simulink model "Swarm_Robot_Final"  (R2020b)
settings: Solver=FixedStepAuto  StartTime=0.0  StopTime=inf  FixedStep=sampleTime  RelTol=1e-3
PreLoadFcn:
  | % Simulation parameters
  | load exampleMap
  | sampleTime = 0.05;
  | 
  | % Robot parameters
  | wheelRadius = 0.025;
  | robotRadius = 0.35;
  | 
  | % Lidar parameters
  | sensorOffset = [0,0];
  | scanAngles = linspace(-pi/2,pi/2,9)';
  | maxRange = 5;
libraries: mobileRoboticsLib x10
settings Model: EnablePacing=on  Creator=scastro  LastModifiedBy=Ashish Sharma
settings DataIOCC: ReturnWorkspaceOutputs=off
settings DebuggingCC: PregeneratedLibrarySubsystemCodeDiagnostic=none  ArithmeticOperatorsInVariantConditions=warning
settings SFSimCC: SimUseLocalCustomCode=off  CustomCodeUndefinedFunction=UseInterfaceOnly
settings RTWCC: RTWUseLocalCustomCode=off

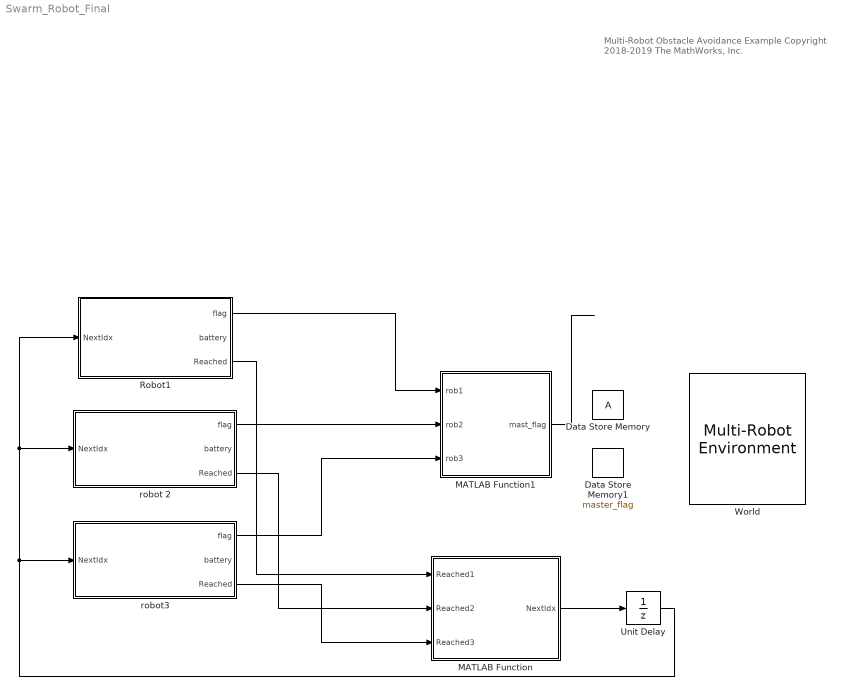
== system Swarm_Robot_Final ==
  note: Multi-Robot Obstacle
      | Avoidance Example
      |
      | Copyright 2018-2019 The MathWorks, Inc.
  Data Store Memory : DataStoreMemory  ReadBeforeWriteMsg=warning  WriteAfterWriteMsg=warning  WriteAfterReadMsg=warning  InitialValue=[1000 1000 1000]  ShowAdditionalParam=off  OutDataTypeStr=double
  Data Store Memory1 : DataStoreMemory  DataStoreName=master_flag  ReadBeforeWriteMsg=warning  WriteAfterWriteMsg=warning  WriteAfterReadMsg=warning  ShowAdditionalParam=off  OutDataTypeStr=double
  MATLAB Function : MATLAB Function  TreatAsAtomicUnit=on
  MATLAB Function1 : MATLAB Function  TreatAsAtomicUnit=on
  "Robot1 " : Subsystem
  Unit Delay : UnitDelay  SampleTime=-1  HasFrameUpgradeWarning=on
  World : mobileRoboticsLib/Environments/Multi-Robot Environment  numRobots=3  showWaypoints=off  showObjects=off  objectColors=[1 0 0;0 1 0;0 0 1]  objectMarkers='s'  showRobotIds=on  plotSensorLines=on
      settings: SourceProductName=Mobile Robotics Simulation Toolbox
  robot 2 : Subsystem
  robot3 : Subsystem
  wires:
  "Robot1 "/1(flag) -> MATLAB Function1/1(rob1)
  robot 2/1(flag) -> MATLAB Function1/2(rob2)
  robot3/1(flag) -> MATLAB Function1/3(rob3)
  "Robot1 "/3(Reached) -> MATLAB Function/1(Reached1)
  MATLAB Function/1(NextIdx) -> Unit Delay/1
  Unit Delay/1 -> "Robot1 "/1(NextIdx), robot 2/1(NextIdx), robot3/1(NextIdx)
  robot 2/3(Reached) -> MATLAB Function/2(Reached2)
  robot3/3(Reached) -> MATLAB Function/3(Reached3)
  MATLAB Function1/1(mast_flag) -> ?

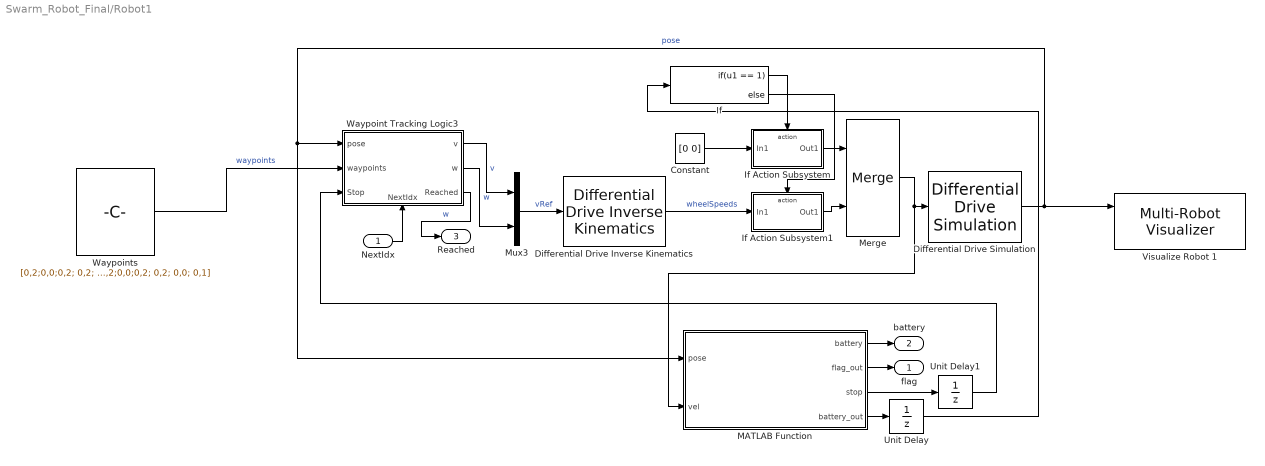
== system Swarm_Robot_Final/Robot1  ==
  NextIdx : Inport
  Constant : Constant  Value=[0 0]
  Differential Drive Inverse Kinematics : mobileRoboticsLib/Kinematic Models/Differential Drive/Differential Drive Inverse Kinematics  wheelRadius=R  wheelBase=L
      settings: SourceProductName=Mobile Robotics Simulation Toolbox
  Differential Drive Simulation : mobileRoboticsLib/Kinematic Models/Differential Drive/Differential Drive Simulation  wheelRadius=R  wheelBase=L  initX=0  initY=2  initAngle=0  Ts=sampleTime
      settings: SourceProductName=Mobile Robotics Simulation Toolbox
  If : If  IfExpression=u1 == 1
  If Action Subsystem : Subsystem  TreatAsAtomicUnit=on
  If Action Subsystem1 : Subsystem  TreatAsAtomicUnit=on
  MATLAB Function : MATLAB Function  TreatAsAtomicUnit=on
  Merge : Merge
  Mux3 : Mux  Inputs=2
  Unit Delay : UnitDelay  SampleTime=-1  HasFrameUpgradeWarning=on
  Unit Delay1 : UnitDelay  SampleTime=-1  HasFrameUpgradeWarning=on
  Visualize Robot 1 : mobileRoboticsLib/Environments/Multi-Robot Visualizer  idx=1  radius=robotRadius  robotColor=[0 0 1]  showTraj=off  hasLidar=on  sensorOffset=sensorOffset  scanAngles=scanAngles  maxNumScans=0  hasObjDetector=off  objDetectorOffset=[0,0]  objDetectorAngle=0  objDetectorFOV=pi/2  objDetectorMaxRange=5  hasRobotDetector=off  robotDetectorOffset=[0,0]  robotDetectorAngle=0  robotDetectorFOV=pi/3  robotDetectorMaxRange=5  robotDetectorNumDetections=0
      settings: SourceProductName=Mobile Robotics Simulation Toolbox
  Waypoint Tracking Logic3 : Stateflow chart  TreatAsAtomicUnit=on
      settings: PortSchema="{\"entries\":[{\"content\":{\"sides\":[{\"content\":{\"connectorIds\":[\"In1\",\"In2\",\"In3\"]},\"type\":\"ConnectorPlacement.EquallySpacedRectSide\",\"uuid\":\"0f37e2f5-7e3e-44b4-b5ad-f9c608efa7e9\"},{\"content\":{\"connectorIds\":[\"Out1\",\"Out2\",\"Out3\"],\"side\":\"RIGHT\"},\"type\":\"ConnectorPlacement.EquallySpacedRectSide\",\"uuid\":\"845bf79f-ea31-423e-b1b0-9ff668e9d8f6\"},{\"content\":{\"connectorIds\":[],\"side\":\"TOP\"},\"type\":\"ConnectorPlacement.EquallySpacedRectSide\",\"uuid\":\"8bec6743-f757-46fc-95b1-a88bb4057338\"},{\"content\":{\"connectorIds\":[\"In4\"],\"side\":\"BOTTOM\"},\"type\":\"ConnectorPlacement.EquallySpacedRectSide\",\"uuid\":\"241e6e67-ff0c-43d0-b4d4-f7a4fa1e9b40\"},{\"content\":{\"connectorIds\":[],\"side\":\"HIDDEN\"},\"type\":\"ConnectorPlacement.EquallySpacedRectSide\",\"uuid\":\"709a4cd5-ab66-4303-a1be-0f54eaafc229\"}]},\"type\":\"ConnectorPlacement.EquallySpacedConnector\",\"uuid\":\"0437a356-16a4-4e9a-ad43-fdf8419276a1\"}],\"packageUris\":[\"http://schema.mathworks.com/mf0/Connector/R2020b\"],\"version\":\"1.0\"}"
  Waypoints : Constant  Value=[0,2;0,0;0,2; 0,2; 0,0; 0,1;0,2;0,0;0,2; 0,2; 0,0; 0,1;0,2;0,0;0,2; 0,2; 0,0; 0,1]
  flag : Outport
  battery : Outport  Port=2
  Reached : Outport  Port=3
  wires:
  Waypoints/1 -> Waypoint Tracking Logic3/2(waypoints)  "waypoints"
  MATLAB Function/1(battery) -> battery/1
  Differential Drive Simulation/1 -> Visualize Robot 1/1, MATLAB Function/1(pose), Waypoint Tracking Logic3/1(pose)  "pose"
  Merge/1 -> MATLAB Function/2(vel), Differential Drive Simulation/1
  Mux3/1 -> Differential Drive Inverse Kinematics/1  "vRef"
  MATLAB Function/2(flag_out) -> flag/1
  If/1 -> If Action Subsystem/Action
  If/2 -> If Action Subsystem1/Action
  Constant/1 -> If Action Subsystem/1(In1)
  If Action Subsystem1/1(Out1) -> Merge/2
  If Action Subsystem/1(Out1) -> Merge/1
  Waypoint Tracking Logic3/1(v) -> Mux3/1  "v"
  Differential Drive Inverse Kinematics/1 -> If Action Subsystem1/1(In1)  "wheelSpeeds"
  Waypoint Tracking Logic3/2(w) -> Mux3/2  "w"
  NextIdx/1 -> Waypoint Tracking Logic3/4(NextIdx)
  Waypoint Tracking Logic3/3(Reached) -> Reached/1  "w"
  MATLAB Function/4(battery_out) -> Unit Delay/1
  Unit Delay/1 -> If/1
  MATLAB Function/3(stop) -> Unit Delay1/1
  Unit Delay1/1 -> Waypoint Tracking Logic3/3(Stop)

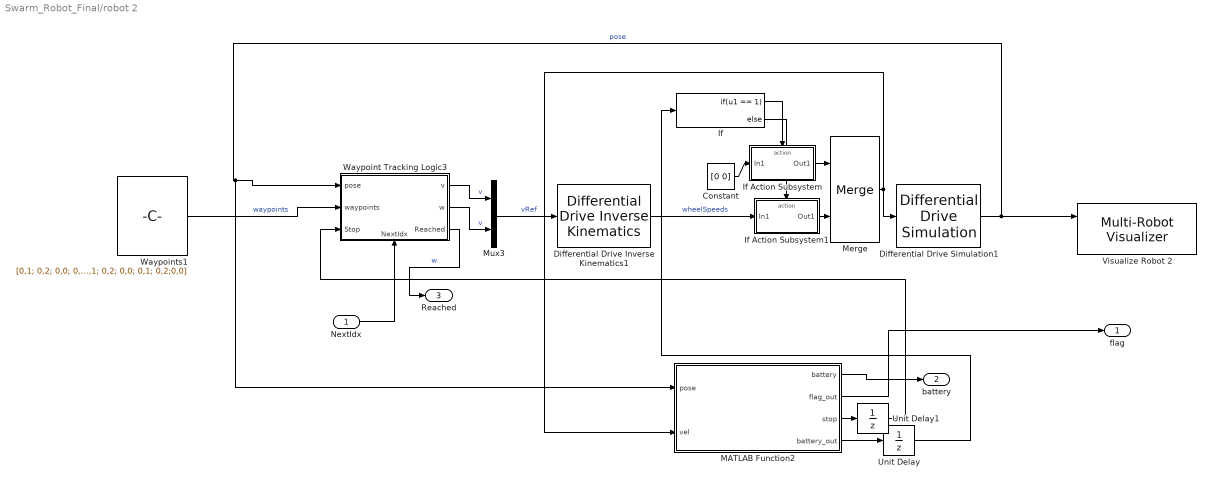
== system Swarm_Robot_Final/robot 2 ==
  NextIdx : Inport
  Constant : Constant  Value=[0 0]
  Differential Drive Inverse Kinematics1 : mobileRoboticsLib/Kinematic Models/Differential Drive/Differential Drive Inverse Kinematics  wheelRadius=R  wheelBase=L
      settings: SourceProductName=Mobile Robotics Simulation Toolbox
  Differential Drive Simulation1 : mobileRoboticsLib/Kinematic Models/Differential Drive/Differential Drive Simulation  wheelRadius=R  wheelBase=L  initX=0  initY=1  initAngle=0  Ts=sampleTime
      settings: SourceProductName=Mobile Robotics Simulation Toolbox
  If : If  IfExpression=u1 == 1
  If Action Subsystem : Subsystem  TreatAsAtomicUnit=on
  If Action Subsystem1 : Subsystem  TreatAsAtomicUnit=on
  MATLAB Function2 : MATLAB Function  TreatAsAtomicUnit=on
  Merge : Merge
  Mux3 : Mux  Inputs=2
  Unit Delay : UnitDelay  SampleTime=-1  HasFrameUpgradeWarning=on
  Unit Delay1 : UnitDelay  SampleTime=-1  HasFrameUpgradeWarning=on
  Visualize Robot 2 : mobileRoboticsLib/Environments/Multi-Robot Visualizer  idx=2  radius=robotRadius  robotColor=[0 0 1]  showTraj=off  hasLidar=on  sensorOffset=sensorOffset  scanAngles=scanAngles  maxNumScans=0  hasObjDetector=off  objDetectorOffset=[0 0]  objDetectorAngle=0  objDetectorFOV=pi/2  objDetectorMaxRange=5  hasRobotDetector=off  robotDetectorOffset=[0,0]  robotDetectorAngle=0  robotDetectorFOV=pi/3  robotDetectorMaxRange=5  robotDetectorNumDetections=0
      settings: SourceProductName=Mobile Robotics Simulation Toolbox
  Waypoint Tracking Logic3 : Stateflow chart  TreatAsAtomicUnit=on
      settings: PortSchema="{\"entries\":[{\"content\":{\"sides\":[{\"content\":{\"connectorIds\":[\"In1\",\"In2\",\"In3\"]},\"type\":\"ConnectorPlacement.EquallySpacedRectSide\",\"uuid\":\"0f37e2f5-7e3e-44b4-b5ad-f9c608efa7e9\"},{\"content\":{\"connectorIds\":[\"Out1\",\"Out2\",\"Out3\"],\"side\":\"RIGHT\"},\"type\":\"ConnectorPlacement.EquallySpacedRectSide\",\"uuid\":\"845bf79f-ea31-423e-b1b0-9ff668e9d8f6\"},{\"content\":{\"connectorIds\":[],\"side\":\"TOP\"},\"type\":\"ConnectorPlacement.EquallySpacedRectSide\",\"uuid\":\"8bec6743-f757-46fc-95b1-a88bb4057338\"},{\"content\":{\"connectorIds\":[\"In4\"],\"side\":\"BOTTOM\"},\"type\":\"ConnectorPlacement.EquallySpacedRectSide\",\"uuid\":\"241e6e67-ff0c-43d0-b4d4-f7a4fa1e9b40\"},{\"content\":{\"connectorIds\":[],\"side\":\"HIDDEN\"},\"type\":\"ConnectorPlacement.EquallySpacedRectSide\",\"uuid\":\"709a4cd5-ab66-4303-a1be-0f54eaafc229\"}]},\"type\":\"ConnectorPlacement.EquallySpacedConnector\",\"uuid\":\"0437a356-16a4-4e9a-ad43-fdf8419276a1\"}],\"packageUris\":[\"http://schema.mathworks.com/mf0/Connector/R2020b\"],\"version\":\"1.0\"}"
  Waypoints1 : Constant  Value=[0,1; 0,2; 0,0; 0,1; 0,2;0,0;0,1; 0,2; 0,0; 0,1; 0,2;0,0;0,1; 0,2; 0,0; 0,1; 0,2;0,0]
  flag : Outport
  battery : Outport  Port=2
  Reached : Outport  Port=3
  wires:
  MATLAB Function2/2(flag_out) -> flag/1
  Differential Drive Inverse Kinematics1/1 -> If Action Subsystem1/1(In1)  "wheelSpeeds"
  Mux3/1 -> Differential Drive Inverse Kinematics1/1  "vRef"
  Waypoints1/1 -> Waypoint Tracking Logic3/2(waypoints)  "waypoints"
  Differential Drive Simulation1/1 -> MATLAB Function2/1(pose), Waypoint Tracking Logic3/1(pose), Visualize Robot 2/1  "pose"
  MATLAB Function2/1(battery) -> battery/1
  If Action Subsystem1/1(Out1) -> Merge/2
  If/2 -> If Action Subsystem1/Action
  Constant/1 -> If Action Subsystem/1(In1)
  If/1 -> If Action Subsystem/Action
  If Action Subsystem/1(Out1) -> Merge/1
  Merge/1 -> Differential Drive Simulation1/1, MATLAB Function2/2(vel)
  NextIdx/1 -> Waypoint Tracking Logic3/4(NextIdx)
  Waypoint Tracking Logic3/1(v) -> Mux3/1  "v"
  Waypoint Tracking Logic3/2(w) -> Mux3/2  "v"
  Waypoint Tracking Logic3/3(Reached) -> Reached/1  "w"
  MATLAB Function2/4(battery_out) -> Unit Delay/1
  Unit Delay/1 -> If/1
  MATLAB Function2/3(stop) -> Unit Delay1/1
  Unit Delay1/1 -> Waypoint Tracking Logic3/3(Stop)

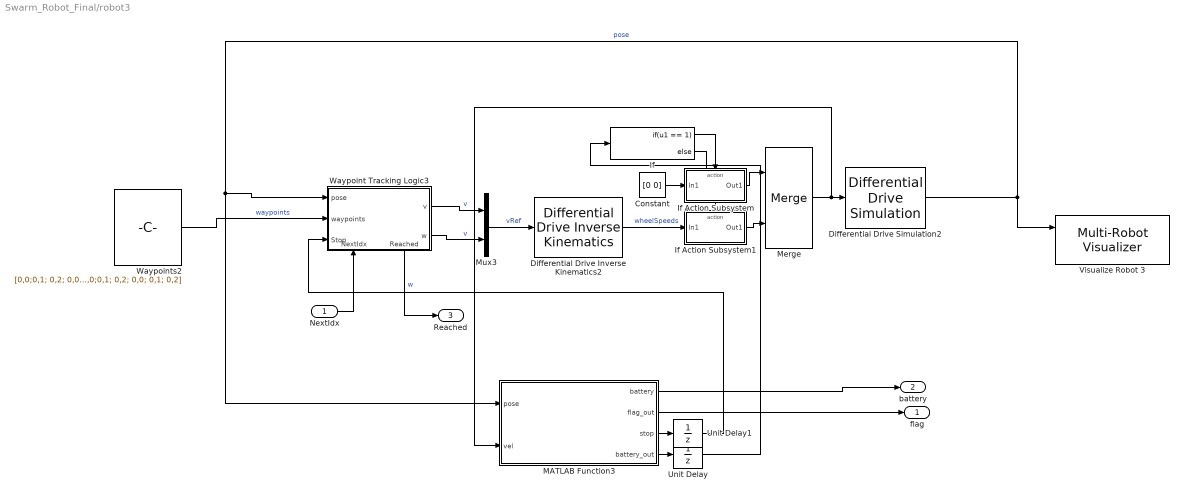
== system Swarm_Robot_Final/robot3 ==
  NextIdx : Inport
  Constant : Constant  Value=[0 0]
  Differential Drive Inverse Kinematics2 : mobileRoboticsLib/Kinematic Models/Differential Drive/Differential Drive Inverse Kinematics  wheelRadius=R  wheelBase=L
      settings: SourceProductName=Mobile Robotics Simulation Toolbox
  Differential Drive Simulation2 : mobileRoboticsLib/Kinematic Models/Differential Drive/Differential Drive Simulation  wheelRadius=R  wheelBase=L  initX=0  initY=0  initAngle=0  Ts=sampleTime
      settings: SourceProductName=Mobile Robotics Simulation Toolbox
  If : If  IfExpression=u1 == 1
  If Action Subsystem : Subsystem  TreatAsAtomicUnit=on
  If Action Subsystem1 : Subsystem  TreatAsAtomicUnit=on
  MATLAB Function3 : MATLAB Function  TreatAsAtomicUnit=on
  Merge : Merge
  Mux3 : Mux  Inputs=2
  Unit Delay : UnitDelay  SampleTime=-1  HasFrameUpgradeWarning=on
  Unit Delay1 : UnitDelay  SampleTime=-1  HasFrameUpgradeWarning=on
  Visualize Robot 3 : mobileRoboticsLib/Environments/Multi-Robot Visualizer  idx=3  radius=robotRadius  robotColor=[0 0 1]  showTraj=off  hasLidar=on  sensorOffset=sensorOffset  scanAngles=scanAngles  maxNumScans=0  hasObjDetector=off  objDetectorOffset=[0 0]  objDetectorAngle=0  objDetectorFOV=pi/2  objDetectorMaxRange=5  hasRobotDetector=off  robotDetectorOffset=[0,0]  robotDetectorAngle=0  robotDetectorFOV=pi/3  robotDetectorMaxRange=5  robotDetectorNumDetections=0
      settings: SourceProductName=Mobile Robotics Simulation Toolbox
  Waypoint Tracking Logic3 : Stateflow chart  TreatAsAtomicUnit=on
      settings: PortSchema="{\"entries\":[{\"content\":{\"sides\":[{\"content\":{\"connectorIds\":[\"In1\",\"In2\",\"In3\"]},\"type\":\"ConnectorPlacement.EquallySpacedRectSide\",\"uuid\":\"0f37e2f5-7e3e-44b4-b5ad-f9c608efa7e9\"},{\"content\":{\"connectorIds\":[\"Out1\",\"Out2\"],\"side\":\"RIGHT\"},\"type\":\"ConnectorPlacement.EquallySpacedRectSide\",\"uuid\":\"845bf79f-ea31-423e-b1b0-9ff668e9d8f6\"},{\"content\":{\"connectorIds\":[],\"side\":\"TOP\"},\"type\":\"ConnectorPlacement.EquallySpacedRectSide\",\"uuid\":\"8bec6743-f757-46fc-95b1-a88bb4057338\"},{\"content\":{\"connectorIds\":[\"In4\",\"Out3\"],\"side\":\"BOTTOM\"},\"type\":\"ConnectorPlacement.EquallySpacedRectSide\",\"uuid\":\"241e6e67-ff0c-43d0-b4d4-f7a4fa1e9b40\"},{\"content\":{\"connectorIds\":[],\"side\":\"HIDDEN\"},\"type\":\"ConnectorPlacement.EquallySpacedRectSide\",\"uuid\":\"709a4cd5-ab66-4303-a1be-0f54eaafc229\"}]},\"type\":\"ConnectorPlacement.EquallySpacedConnector\",\"uuid\":\"0437a356-16a4-4e9a-ad43-fdf8419276a1\"}],\"packageUris\":[\"http://schema.mathworks.com/mf0/Connector/R2020b\"],\"version\":\"1.0\"}"
  Waypoints2 : Constant  Value=[0,0;0,1; 0,2; 0,0; 0,1; 0,2;0,0;0,1; 0,2; 0,0; 0,1; 0,2;0,0;0,1; 0,2; 0,0; 0,1; 0,2]
  flag : Outport
  battery : Outport  Port=2
  Reached : Outport  Port=3
  wires:
  MATLAB Function3/2(flag_out) -> flag/1
  Differential Drive Simulation2/1 -> Visualize Robot 3/1, MATLAB Function3/1(pose), Waypoint Tracking Logic3/1(pose)  "pose"
  Waypoints2/1 -> Waypoint Tracking Logic3/2(waypoints)  "waypoints"
  Mux3/1 -> Differential Drive Inverse Kinematics2/1  "vRef"
  Differential Drive Inverse Kinematics2/1 -> If Action Subsystem1/1(In1)  "wheelSpeeds"
  MATLAB Function3/1(battery) -> battery/1
  If Action Subsystem1/1(Out1) -> Merge/2
  If/2 -> If Action Subsystem1/Action
  Constant/1 -> If Action Subsystem/1(In1)
  If/1 -> If Action Subsystem/Action
  If Action Subsystem/1(Out1) -> Merge/1
  Merge/1 -> MATLAB Function3/2(vel), Differential Drive Simulation2/1
  NextIdx/1 -> Waypoint Tracking Logic3/4(NextIdx)
  Waypoint Tracking Logic3/1(v) -> Mux3/1  "v"
  Waypoint Tracking Logic3/2(w) -> Mux3/2  "v"
  Waypoint Tracking Logic3/3(Reached) -> Reached/1  "w"
  MATLAB Function3/4(battery_out) -> Unit Delay/1
  Unit Delay/1 -> If/1
  MATLAB Function3/3(stop) -> Unit Delay1/1
  Unit Delay1/1 -> Waypoint Tracking Logic3/3(Stop)

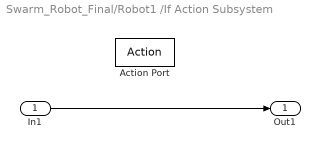
== system Swarm_Robot_Final/Robot1 /If Action Subsystem ==
  In1 : Inport
  Action Port : ActionPort  ActionPortLabel=if(u1 == 1)
  Out1 : Outport
  wires:
  In1/1 -> Out1/1

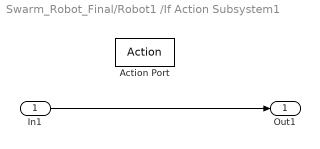
== system Swarm_Robot_Final/Robot1 /If Action Subsystem1 ==
  In1 : Inport
  Action Port : ActionPort  ActionPortLabel=else
  Out1 : Outport
  wires:
  In1/1 -> Out1/1

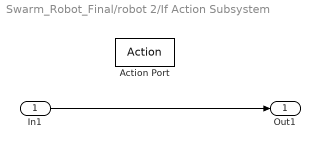
== system Swarm_Robot_Final/robot 2/If Action Subsystem ==
  In1 : Inport
  Action Port : ActionPort  ActionPortLabel=if(u1 == 1)
  Out1 : Outport
  wires:
  In1/1 -> Out1/1

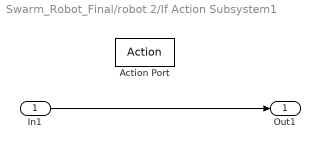
== system Swarm_Robot_Final/robot 2/If Action Subsystem1 ==
  In1 : Inport
  Action Port : ActionPort  ActionPortLabel=else
  Out1 : Outport
  wires:
  In1/1 -> Out1/1

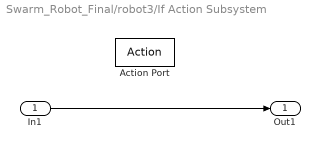
== system Swarm_Robot_Final/robot3/If Action Subsystem ==
  In1 : Inport
  Action Port : ActionPort  ActionPortLabel=if(u1 == 1)
  Out1 : Outport
  wires:
  In1/1 -> Out1/1

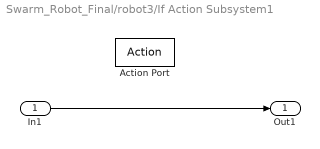
== system Swarm_Robot_Final/robot3/If Action Subsystem1 ==
  In1 : Inport
  Action Port : ActionPort  ActionPortLabel=else
  Out1 : Outport
  wires:
  In1/1 -> Out1/1

== matlab function Swarm_Robot_Final/robot 2/MATLAB Function2 ==
  data: battery output; pose input; flag_out output; A data_store_memory; stop output; master_flag data_store_memory; battery_out output; vel input
function [battery, flag_out,stop, battery_out]  = battery( pose,vel) 
home = [0.1,0.1,0]';
global A;
global master_flag;
charge = 4;
discharge =2;
battery = A(2);
stop=0;
battery_out=0;
if(abs(pose(2)))<home(2) 
    flag_out = 1;
    battery = battery +charge;
    if battery>500
        flag_out=0;
    end
else
    flag_out =0;
end

if vel(1)>0 || vel(2)>0
    battery= battery-discharge;
end 
if  master_flag==1 
    stop=1;
end

if battery<0 
    battery_out=1;
end
A(2) = battery;

== matlab function Swarm_Robot_Final/robot3/MATLAB Function3 ==
  data: pose input; battery output; vel input; flag_out output; A data_store_memory; stop output; master_flag data_store_memory; battery_out output
function [battery, flag_out,stop, battery_out]  = battery( pose, vel) 
home = [0.1,0.1,0]';
global A;
global master_flag;
charge = 4;
discharge =2;
battery = A(3);
stop=0;
battery_out=0;


if(abs(pose(2)))<home(2)  
    flag_out = 1;
    battery = battery +charge;
    if battery>500
        flag_out=0;
    end
else
    flag_out =0;
end

if vel(1)>0 || vel(2)>0
    battery= battery-discharge;
end 
if  master_flag==1 
    stop=1;
end

if battery<0 
    battery_out=1;
end
A(3) = battery;

== stateflow chart Swarm_Robot_Final/robot 2/Waypoint Tracking Logic3 ==
  state StopEntry
    entry:
    v =0;
    w=0;
  state FollowWaypoints
    entry:
    goalPoint = waypoints(idx,:);
    entry, during:
    [angle,range] = trackGoal(goalPoint);
    Reached=false;
    (default) -> (junction 20)
    FollowWaypoints -> (junction 20) [order 1]
    (junction 20) -> (junction 24) [order 1] : % Set angular speed if
        | % angle outside deadband
        | [abs(angle) > pi/24]
    (junction 20) -> (junction 30) [order 2] : {w = 0;}
    (junction 24) -> (junction 49) : % Proportional
        | % control
        | {w = 1.5*angle;}
    (junction 49) -> (junction 30)
  state ReachedGoal
    entry:
    v = 0;
    w = 0.5;
  state NextIdxEntry
    entry:
    v=0;
    w=0;
  (default) -> FollowWaypoints : {
      | v = 0.5;
      | idx = 1;
      | numPts = size(waypoints,1);
      | Reached=false;
      | }
  StopEntry -> (junction 67) : [Stop==0]
  (junction 67) -> FollowWaypoints : {v=0.5}
  (junction 39) -> StopEntry [order 1] : [Stop==1]
  FollowWaypoints -> (junction 71) [order 1] : % Check if goal reached
      | [range < 0.1]
  (junction 71) -> (junction 39)
  (junction 39) -> ReachedGoal [order 2] : % Stop if final waypoint
      | [idx == numPts]
  (junction 39) -> NextIdxEntry [order 3] : {Reached =true;}
  NextIdxEntry -> (junction 42) : [NextIdx==true]
  (junction 42) -> FollowWaypoints : % Go to the next waypoint
      | {idx = idx + 1;
      | v=0.5;}
  data: goal function_input; ang function_output; dist function_output; pose input; waypoints input; v output; w output; angle local; range local; idx local; numPts local; goalPoint local; Stop input; Reached output boolean; NextIdx input
  function [ang,dist] = trackGoal(goal):
    | function [ang,dist] = trackGoal(goal)
    | % Finds the angle (theta) and distance (dist) between the 
    | % vehicle and a goal point
    |     
    | posDiff = [goal(1)-pose(1);goal(2)-pose(2)];
    | 
    | ang = angdiff(pose(3),atan2(posDiff(2),posDiff(1)));
    | dist = sqrt(posDiff(1)^2 + posDiff(2)^2);

== stateflow chart Swarm_Robot_Final/robot3/Waypoint Tracking Logic3 ==
  state StopEntry
    entry:
    v =0;
    w=0;
  state FollowWaypoints
    entry:
    goalPoint = waypoints(idx,:);
    entry, during:
    [angle,range] = trackGoal(goalPoint);
    Reached=false;
    (default) -> (junction 20)
    FollowWaypoints -> (junction 20) [order 1]
    (junction 20) -> (junction 24) [order 1] : % Set angular speed if
        | % angle outside deadband
        | [abs(angle) > pi/24]
    (junction 20) -> (junction 30) [order 2] : {w = 0;}
    (junction 24) -> (junction 49) : % Proportional
        | % control
        | {w = 1.5*angle;}
    (junction 49) -> (junction 30)
  state ReachedGoal
    entry:
    v = 0;
    w = 0.5;
  state NextIdxEntry
    entry:
    v=0;
    w=0;
  (default) -> FollowWaypoints : {
      | v = 0.5;
      | idx = 1;
      | numPts = size(waypoints,1);
      | Reached=false;
      | }
  StopEntry -> (junction 67) : [Stop==0]
  (junction 67) -> FollowWaypoints : {v=0.5}
  (junction 39) -> StopEntry [order 1] : [Stop==1]
  FollowWaypoints -> (junction 71) [order 1] : % Check if goal reached
      | [range < 0.1]
  (junction 71) -> (junction 39)
  (junction 39) -> ReachedGoal [order 2] : % Stop if final waypoint
      | [idx == numPts]
  (junction 39) -> NextIdxEntry [order 3] : {Reached =true;}
  NextIdxEntry -> (junction 42) : [NextIdx==true]
  (junction 42) -> FollowWaypoints : % Go to the next waypoint
      | {idx = idx + 1;
      | v=0.5;}
  data: goal function_input; ang function_output; dist function_output; pose input; waypoints input; v output; w output; angle local; range local; idx local; numPts local; goalPoint local; Stop input; Reached output boolean; NextIdx input
  function [ang,dist] = trackGoal(goal):
    | function [ang,dist] = trackGoal(goal)
    | % Finds the angle (theta) and distance (dist) between the 
    | % vehicle and a goal point
    |     
    | posDiff = [goal(1)-pose(1);goal(2)-pose(2)];
    | 
    | ang = angdiff(pose(3),atan2(posDiff(2),posDiff(1)));
    | dist = sqrt(posDiff(1)^2 + posDiff(2)^2);

== stateflow chart Swarm_Robot_Final/Robot1 /Waypoint Tracking Logic3 ==
  state StopEntry
    entry:
    v =0;
    w=0;
  state FollowWaypoints
    entry:
    goalPoint = waypoints(idx,:);
    entry, during:
    [angle,range] = trackGoal(goalPoint);
    Reached=false;
    (default) -> (junction 20)
    FollowWaypoints -> (junction 20) [order 1]
    (junction 20) -> (junction 24) [order 1] : % Set angular speed if
        | % angle outside deadband
        | [abs(angle) > pi/24]
    (junction 20) -> (junction 30) [order 2] : {w = 0;}
    (junction 24) -> (junction 49) : % Proportional
        | % control
        | {w = 1.5*angle;}
    (junction 49) -> (junction 30)
  state ReachedGoal
    entry:
    v = 0;
    w = 0.5;
  state NextIdxEntry
    entry:
    v=0;
    w=0;
  (default) -> FollowWaypoints : {
      | v = 0.5;
      | idx = 1;
      | numPts = size(waypoints,1);
      | Reached=false;
      | }
  StopEntry -> (junction 67) : [Stop==0]
  (junction 67) -> FollowWaypoints : {v=0.5}
  (junction 39) -> StopEntry [order 1] : [Stop==1]
  FollowWaypoints -> (junction 71) [order 1] : % Check if goal reached
      | [range < 0.1]
  (junction 71) -> (junction 39)
  (junction 39) -> ReachedGoal [order 2] : % Stop if final waypoint
      | [idx == numPts]
  (junction 39) -> NextIdxEntry [order 3] : {Reached =true;}
  NextIdxEntry -> (junction 42) : [NextIdx==true]
  (junction 42) -> FollowWaypoints : % Go to the next waypoint
      | {idx = idx + 1;
      | v=0.5;}
  data: goal function_input; ang function_output; dist function_output; pose input; waypoints input; v output; w output; angle local; range local; idx local; numPts local; goalPoint local; Stop input; Reached output boolean; NextIdx input
  function [ang,dist] = trackGoal(goal):
    | function [ang,dist] = trackGoal(goal)
    | % Finds the angle (theta) and distance (dist) between the 
    | % vehicle and a goal point
    |     
    | posDiff = [goal(1)-pose(1);goal(2)-pose(2)];
    | 
    | ang = angdiff(pose(3),atan2(posDiff(2),posDiff(1)));
    | dist = sqrt(posDiff(1)^2 + posDiff(2)^2);

== matlab function Swarm_Robot_Final/MATLAB Function ==
  data: Reached1 input; NextIdx output; Reached2 input; Reached3 input
function NextIdx= NextIdx_fcn(Reached1, Reached2, Reached3)
if Reached1==true && Reached2==true && Reached3==true
    NextIdx=true;
else
    NextIdx=false;
end

== matlab function Swarm_Robot_Final/MATLAB Function1 ==
  data: rob1 input; rob2 input; rob3 input; master_flag data_store_memory; mast_flag output
function mast_flag = branch_manager(rob1,rob2,rob3)
flags=[rob1,rob2,rob3];
global master_flag;
if rob1==1 || rob2==1 || rob3==1
    master_flag=1;
else
    master_flag=0;
end
mast_flag=master_flag;

== matlab function Swarm_Robot_Final/Robot1 /MATLAB Function ==
  data: battery output; pose input; flag_out output; A data_store_memory; stop output size=1; master_flag data_store_memory; battery_out output; vel input
function [battery, flag_out,stop, battery_out]  = battery( pose,vel) 
home = [0.1,0.2,0]';
global A;
global master_flag;
charge = 4;
discharge =2;
battery = A(1);
stop=0;
battery_out=0;

if(abs(pose(2)))<home(2)
    flag_out = 1;
    battery = battery +charge;
    if battery>500
        flag_out=0;
    end
else
    flag_out =0;
end

if vel(1)>0 || vel(2)>0
    battery= battery-discharge;
end 

if  master_flag==1 
    stop=1;
end

if battery<0 
    battery_out=1;
end
A(1) = battery;
